simulink model "SWC_HALOUT_type"  (R2021b)
settings: Solver=FixedStepDiscrete  StartTime=0.0  StopTime=10.0  FixedStep=0.005  RelTol=1e-3
values from neighbouring files (symbols this model uses):
  DTC_10020B = Simulink.Parameter    [DTC_Constant_Definition.m]
  DTC_10020C = Simulink.Parameter    [DTC_Constant_Definition.m]
  DTC_10020D = Simulink.Parameter    [DTC_Constant_Definition.m]
  DTC_10020E = Simulink.Parameter    [DTC_Constant_Definition.m]
  DTC_100210 = Simulink.Parameter    [DTC_Constant_Definition.m]
  DTC_100211 = Simulink.Parameter    [DTC_Constant_Definition.m]
  DTC_100212 = Simulink.Parameter    [DTC_Constant_Definition.m]
  DTC_100213 = Simulink.Parameter    [DTC_Constant_Definition.m]
  DTC_100214 = Simulink.Parameter    [DTC_Constant_Definition.m]
  DTC_100215 = Simulink.Parameter    [DTC_Constant_Definition.m]
  DTC_100216 = Simulink.Parameter    [DTC_Constant_Definition.m]
  DTC_100217 = Simulink.Parameter    [DTC_Constant_Definition.m]
  DTC_100218 = Simulink.Parameter    [DTC_Constant_Definition.m]
  DTC_100219 = Simulink.Parameter    [DTC_Constant_Definition.m]
  DTC_10021A = Simulink.Parameter    [DTC_Constant_Definition.m]
  DTC_10021B = Simulink.Parameter    [DTC_Constant_Definition.m]
  DTC_10021C = Simulink.Parameter    [DTC_Constant_Definition.m]
  DTC_10021D = Simulink.Parameter    [DTC_Constant_Definition.m]
  DTC_10021E = Simulink.Parameter    [DTC_Constant_Definition.m]
  DTC_100220 = Simulink.Parameter    [DTC_Constant_Definition.m]
  DTC_100221 = Simulink.Parameter    [DTC_Constant_Definition.m]
  DTC_100223 = Simulink.Parameter    [DTC_Constant_Definition.m]
  DTC_100224 = Simulink.Parameter    [DTC_Constant_Definition.m]
  DTC_100225 = Simulink.Parameter    [DTC_Constant_Definition.m]
  DTC_100226 = Simulink.Parameter    [DTC_Constant_Definition.m]
  DTC_100227 = Simulink.Parameter    [DTC_Constant_Definition.m]
  DTC_100242 = Simulink.Parameter    [DTC_Constant_Definition.m]
  DTC_100243 = Simulink.Parameter    [DTC_Constant_Definition.m]
  DTC_100244 = Simulink.Parameter    [DTC_Constant_Definition.m]
  DTC_100247 = Simulink.Parameter    [DTC_Constant_Definition.m]
  DTC_100248 = Simulink.Parameter    [DTC_Constant_Definition.m]
  DTC_100249 = Simulink.Parameter    [DTC_Constant_Definition.m]
  DTC_100250 = Simulink.Parameter    [DTC_Constant_Definition.m]
  DTC_100251 = Simulink.Parameter    [DTC_Constant_Definition.m]
  DTC_100252 = Simulink.Parameter    [DTC_Constant_Definition.m]
  DTC_100A10 = Simulink.Parameter    [DTC_Constant_Definition.m]
  DTC_100A12 = Simulink.Parameter    [DTC_Constant_Definition.m]
  DTC_100A16 = Simulink.Parameter    [DTC_Constant_Definition.m]
  DTC_100A17 = Simulink.Parameter    [DTC_Constant_Definition.m]
  DTC_100A18 = Simulink.Parameter    [DTC_Constant_Definition.m]
  DTC_100A19 = Simulink.Parameter    [DTC_Constant_Definition.m]
  DTC_500B01 = Simulink.Parameter    [DTC_Constant_Definition.m]
  DTC_500B02 = Simulink.Parameter    [DTC_Constant_Definition.m]
  DTC_500B03 = Simulink.Parameter    [DTC_Constant_Definition.m]
  DTC_500B04 = Simulink.Parameter    [DTC_Constant_Definition.m]
  DTC_500B05 = Simulink.Parameter    [DTC_Constant_Definition.m]
  DTC_500B06 = Simulink.Parameter    [DTC_Constant_Definition.m]
  DTC_500B07 = Simulink.Parameter    [DTC_Constant_Definition.m]
  DTC_500B08 = Simulink.Parameter    [DTC_Constant_Definition.m]
  DTC_500B09 = Simulink.Parameter    [DTC_Constant_Definition.m]
  DTC_500B0A = Simulink.Parameter    [DTC_Constant_Definition.m]
  DTC_500B0B = Simulink.Parameter    [DTC_Constant_Definition.m]
  DTC_500B0C = Simulink.Parameter    [DTC_Constant_Definition.m]
  DTC_500B0D = Simulink.Parameter    [DTC_Constant_Definition.m]
  DTC_500B0E = Simulink.Parameter    [DTC_Constant_Definition.m]
  DTC_500B0F = Simulink.Parameter    [DTC_Constant_Definition.m]
  DTC_500B10 = Simulink.Parameter    [DTC_Constant_Definition.m]
  DTC_90021F = Simulink.Parameter    [DTC_Constant_Definition.m]
  DTC_90022F = Simulink.Parameter    [DTC_Constant_Definition.m]
  DTC_900253 = Simulink.Parameter    [DTC_Constant_Definition.m]
  DTC_900254 = Simulink.Parameter    [DTC_Constant_Definition.m]
  DTC_900301 = Simulink.Parameter    [DTC_Constant_Definition.m]
  DTC_900302 = Simulink.Parameter    [DTC_Constant_Definition.m]
  DTC_900303 = Simulink.Parameter    [DTC_Constant_Definition.m]
  DTC_900304 = Simulink.Parameter    [DTC_Constant_Definition.m]
  DTC_900305 = Simulink.Parameter    [DTC_Constant_Definition.m]
  DTC_900909 = Simulink.Parameter    [DTC_Constant_Definition.m]
  DTC_90090A = Simulink.Parameter    [DTC_Constant_Definition.m]
  DTC_90090B = Simulink.Parameter    [DTC_Constant_Definition.m]
  DTC_90090C = Simulink.Parameter    [DTC_Constant_Definition.m]
  DTC_90090D = Simulink.Parameter    [DTC_Constant_Definition.m]
  DTC_90090E = Simulink.Parameter    [DTC_Constant_Definition.m]
  DTC_90090F = Simulink.Parameter    [DTC_Constant_Definition.m]
  DTC_900910 = Simulink.Parameter    [DTC_Constant_Definition.m]
  DTC_900911 = Simulink.Parameter    [DTC_Constant_Definition.m]
  DTC_900912 = Simulink.Parameter    [DTC_Constant_Definition.m]
  DTC_900913 = Simulink.Parameter    [DTC_Constant_Definition.m]
  DTC_900914 = Simulink.Parameter    [DTC_Constant_Definition.m]
  DTC_C0288F = Simulink.Parameter    [DTC_Constant_Definition.m]
  DTC_C0378F = Simulink.Parameter    [DTC_Constant_Definition.m]
  DTC_C0468F = Simulink.Parameter    [DTC_Constant_Definition.m]
  DTC_C0558F = Simulink.Parameter    [DTC_Constant_Definition.m]
  DTC_C0648F = Simulink.Parameter    [DTC_Constant_Definition.m]
  DTC_C0808F = Simulink.Parameter    [DTC_Constant_Definition.m]
  DTC_D00201 = Simulink.Parameter    [DTC_Constant_Definition.m]
  DTC_D00202 = Simulink.Parameter    [DTC_Constant_Definition.m]
  DTC_D00203 = Simulink.Parameter    [DTC_Constant_Definition.m]
  DTC_D00204 = Simulink.Parameter    [DTC_Constant_Definition.m]
  DTC_D00205 = Simulink.Parameter    [DTC_Constant_Definition.m]
  DTC_D00206 = Simulink.Parameter    [DTC_Constant_Definition.m]
  DTC_D00207 = Simulink.Parameter    [DTC_Constant_Definition.m]
  DTC_D00208 = Simulink.Parameter    [DTC_Constant_Definition.m]
  DTC_D00209 = Simulink.Parameter    [DTC_Constant_Definition.m]
  DTC_D0020A = Simulink.Parameter    [DTC_Constant_Definition.m]
  DTC_D00228 = Simulink.Parameter    [DTC_Constant_Definition.m]
  DTC_D00229 = Simulink.Parameter    [DTC_Constant_Definition.m]
  DTC_D0022A = Simulink.Parameter    [DTC_Constant_Definition.m]
  DTC_D0022B = Simulink.Parameter    [DTC_Constant_Definition.m]
  DTC_D0022C = Simulink.Parameter    [DTC_Constant_Definition.m]
  DTC_D0022D = Simulink.Parameter    [DTC_Constant_Definition.m]
  DTC_D00230 = Simulink.Parameter    [DTC_Constant_Definition.m]
  DTC_D00231 = Simulink.Parameter    [DTC_Constant_Definition.m]
  DTC_D00232 = Simulink.Parameter    [DTC_Constant_Definition.m]
  DTC_D00234 = Simulink.Parameter    [DTC_Constant_Definition.m]
  DTC_D00235 = Simulink.Parameter    [DTC_Constant_Definition.m]
  DTC_D00236 = Simulink.Parameter    [DTC_Constant_Definition.m]
  DTC_D00237 = Simulink.Parameter    [DTC_Constant_Definition.m]
  DTC_D00238 = Simulink.Parameter    [DTC_Constant_Definition.m]
  DTC_D0023A = Simulink.Parameter    [DTC_Constant_Definition.m]
  DTC_D0023B = Simulink.Parameter    [DTC_Constant_Definition.m]
  DTC_D0023C = Simulink.Parameter    [DTC_Constant_Definition.m]
  DTC_D0023D = Simulink.Parameter    [DTC_Constant_Definition.m]
  DTC_D0023E = Simulink.Parameter    [DTC_Constant_Definition.m]
  DTC_D00240 = Simulink.Parameter    [DTC_Constant_Definition.m]
  DTC_D00241 = Simulink.Parameter    [DTC_Constant_Definition.m]
undefined symbols (not defined in the file or in its folder): DIDLen_APPD, DIDLen_APPE, DIDLen_APPPedalZP, DIDLen_APSFunConfig, DIDLen_AutoLock, DIDLen_AutoWipHSpdEN, DIDLen_CALID, DIDLen_CDEODT, DIDLen_CLRDIST, DIDLen_DKCBLESta, DIDLen_DKCKey, DIDLen_DKCSta, DIDLen_DoorNFCAnchorSta, DIDLen_DRLDis, DIDLen_DynoMode, DIDLen_ECUNAME, DIDLen_FDDKCCoordXY, DIDLen_FMHTimer, DIDLen_LFLowPresThre, DIDLen_LFSensorID, DIDLen_LIDAAnchorSta, DIDLen_LRLowPresThre, DIDLen_LRSensorID, DIDLen_MILDIST, DIDLen_NUMPSATRIPSFLTMEMCLR, DIDLen_NVMPedalZP, DIDLen_OBDReq, DIDLen_ODOMETER, DIDLen_PKE, DIDLen_ProtocolId, DIDLen_PSA, DIDLen_QTYPSATRIPS, DIDLen_RFLowPresThre, DIDLen_RFSensorID, DIDLen_RRLowPresThre, DIDLen_RRSensorID, DIDLen_RUNTM, DIDLen_SensorMode, DIDLen_TestGroup, DIDLen_TireSize, DIDLen_TPMSLearnSta, DIDLen_UIDSta, DIDLen_USSConfig, DIDLen_UWBAnchorSta, DIDLen_VIN, DIDLen_VSS, DIDLen_WhlPres, DIDLen_WhlSensorBattSta, DIDLen_WhlTmp, DIDLen_WipRLSCmdCutFilter, DIDLen_WipRLSCmdHoldFilter, DIDLen_XWDMode, DIDNum_APPD, DIDNum_APPE, DIDNum_APPPedalZP, DIDNum_APSFunConfig, DIDNum_AutoLock, DIDNum_AutoWipHSpdEN, DIDNum_CALID, DIDNum_CDEODT ... (+281)
libraries: simulink x213, FVT_lib x160, hdlsllib x6, hcu_lib x5, halout x1
(part 1 of 9)
settings Model: DataDictionary=APPTypes.sldd  Creator=FVT23010  LastModifiedBy=FVT23033
settings DataIOCC: SaveFormat=StructureWithTime
settings OptimizationCC: DefaultParameterBehavior=Inlined  EnhancedBackFolding=on  PassReuseOutputArgsAs=Individual arguments  ZeroExternalMemoryAtStartup=off  ZeroInternalMemoryAtStartup=off  OptimizeBlockOrder=speed  DifferentSizesBufferReuse=on  OptimizationCustomize=off  EfficientTunableParamExpr=on
settings DebuggingCC: ParameterTunabilityLossMsg=error
settings HardwareCC: ProdBitPerPointer=32  ProdBitPerSizeT=32  ProdBitPerPtrDiffT=32  ProdLargestAtomicInteger=Long  ProdLargestAtomicFloat=Double  ProdWordSize=32  ProdLongLongMode=on  ProdHWDeviceType=ARM Compatible->ARM Cortex-M
settings ModelReferenceCC: ModelReferenceNumInstancesAllowed=Single
settings SFSimCC: MATLABDynamicMemAlloc=off
settings RTWCC: Description=AUTOSAR  SystemTargetFile=autosar.tlc  GenCodeOnly=on  TemplateMakefile=ert_default_tmf  PortableWordSizes=on
settings CodeAppCC: ForceParamTrailComments=on  IgnoreCustomStorageClasses=off  OperatorAnnotations=on  SimulinkDataObjDesc=on  SFDataObjDesc=on  InsertBlockDesc=on
settings STFCustomTargetCC: TargetLangStandard=C99 (ISO)  UtilityFuncGeneration=Shared location  MultiwordLength=256  ParMdlRefBuildCompliant=on  CompOptLevelCompliant=on  IncludeMdlTerminateFcn=off  CombineOutputUpdateFcns=on  SuppressErrorStatus=on  ERTCustomFileBanners=on  SupportNonFinite=off  SupportComplex=off  SupportContinuousTime=off  SupportNonInlinedSFcns=off  RemoveResetFunc=on  MATLABClassNameForMDSCustomization=Simulink.SoftwareTarget.ERTCustomization  AutosarCompliant=on  GRTInterface=off  UseToolchainInfoCompliant=on  GenerateSharedConstants=off  LookupTableObjectStructAxisOrder=2,1,3,4,...  LUTObjectStructOrderEvenSpacing=Size,Table,Breakpoints  SystemTargetFile=autosar.tlc
settings ERTTargetCC: TargetLangStandard=C99 (ISO)  UtilityFuncGeneration=Shared location  ConcurrentExecutionCompliant=off  IncludeMdlTerminateFcn=off  SuppressErrorStatus=on  SupportNonFinite=off  SupportComplex=off  ModelStepFunctionPrototypeControlCompliant=off  CPPClassGenCompliant=off  AutosarCompliant=on  GenerateSharedConstants=off  LookupTableObjectStructAxisOrder=2,1,3,4,...  LUTObjectStructOrderEvenSpacing=Size,Table,Breakpoints  GenerateASAP2=on  InlinedParameterPlacement=NonHierarchical  ERTCustomFileTemplate=example_file_process.tlc  ConvertIfToSwitch=off  SuppressUnreachableDefaultCases=off  BooleanTrueId=true_MatlabRTW  BooleanFalseId=false_MatlabRTW

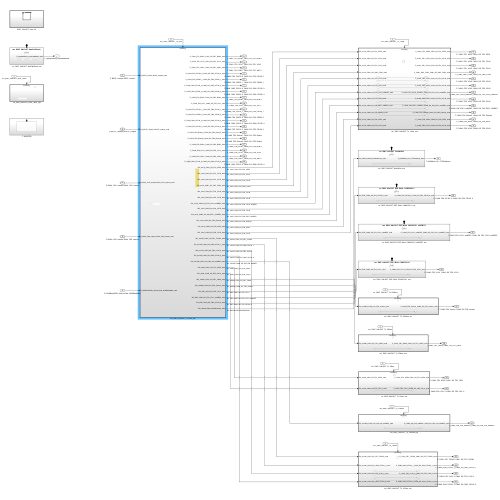
[thumbnail: Simulink's stored preview of the top-level diagram]
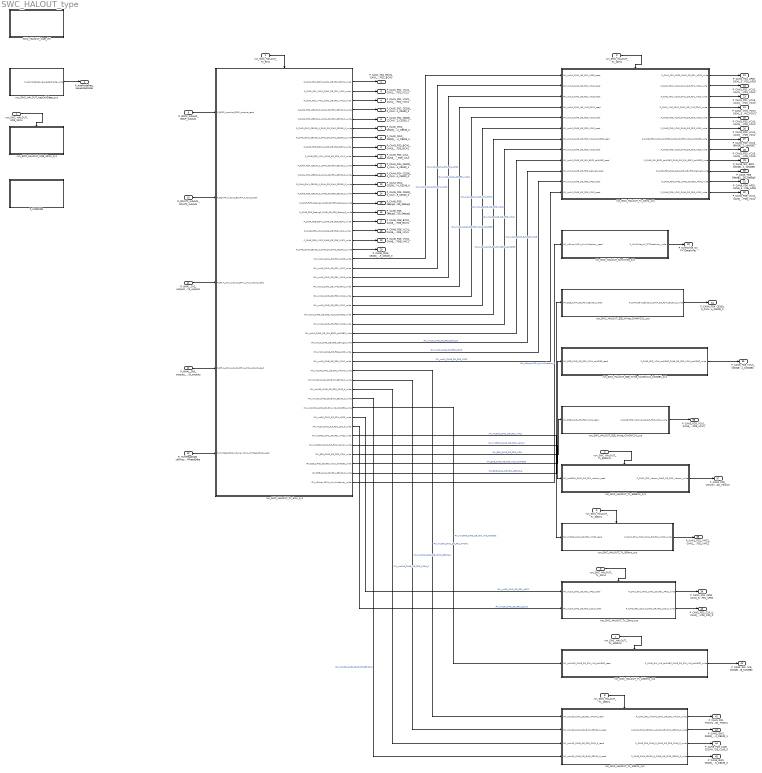
== system SWC_HALOUT_type ==
  run_SWC_HALOUT_UDS_10ms : Inport  SampleTime=0.01  OutputFunctionCall=on
  run_SWC_HALOUT_Tx_5ms : Inport  Port=2  SampleTime=0.005  OutputFunctionCall=on
  run_SWC_HALOUT_Tx_10ms : Inport  Port=3  SampleTime=0.01  OutputFunctionCall=on
  run_SWC_HALOUT_Tx_5000ms : Inport  Port=4  SampleTime=5  OutputFunctionCall=on
  run_SWC_HALOUT_Tx_500ms : Inport  Port=5  SampleTime=0.5  OutputFunctionCall=on
  run_SWC_HALOUT_Tx_20ms : Inport  Port=6  SampleTime=0.02  OutputFunctionCall=on
  run_SWC_HALOUT_Tx_1000ms : Inport  Port=7  SampleTime=1  OutputFunctionCall=on
  run_SWC_HALOUT_Tx_100ms : Inport  Port=8  SampleTime=0.1  OutputFunctionCall=on
  R_BSCP_outputs_BSCP_outputs : Inport  Port=9  OutDataTypeStr=Bus: BSCP_outputs  PortDimensions=1  BusOutputAsStruct=on
  R_BOUTP_outputs_BOUTP_outputs : Inport  Port=10  OutDataTypeStr=Bus: BOUTP_outputs  PortDimensions=1  BusOutputAsStruct=on
  R_BHAL_SYS_outputs_BHAL_SYS_outputs : Inport  Port=11  OutDataTypeStr=Bus: BHAL_SYS_outputs  PortDimensions=1  BusOutputAsStruct=on
  R_BHAL_DID_outputs_BHAL_DID_outputs : Inport  Port=12  OutDataTypeStr=Bus: BHAL_DID_outputs  PortDimensions=1  BusOutputAsStruct=on
  R_NVMReadCDD_u8Array1024_NVMReadData : Inport  Port=13  OutDataTypeStr=uint8  PortDimensions=1024
  P_WDGCDD : Subsystem
  SWC_HALOUT_type_Init : Subsystem
  run_SWC_HALOUT_AppCallSleep_sys : Subsystem
  run_SWC_HALOUT_E2E_Write_CAN3VCU1_sys : Subsystem
  run_SWC_HALOUT_E2E_Write_CAN3VCU1_toNIDEC_sys : Subsystem
  run_SWC_HALOUT_E2E_Write_CAN4VCU1_sys : Subsystem
  run_SWC_HALOUT_NvmWrite_sys : Subsystem
  run_SWC_HALOUT_Tx_1000ms_sys : Subsystem
  run_SWC_HALOUT_Tx_100ms_sys : Subsystem
  run_SWC_HALOUT_Tx_10ms_sys : Subsystem
  run_SWC_HALOUT_Tx_20ms_sys : Subsystem
  run_SWC_HALOUT_Tx_5000ms_sys : Subsystem
  run_SWC_HALOUT_Tx_500ms_sys : Subsystem
  run_SWC_HALOUT_Tx_5ms_sys : Subsystem
  run_SWC_HALOUT_UDS_10ms_sys : Subsystem
  P_AppModeReq_requestedMode : Outport  OutDataTypeStr=Enum: AppModeRequestType  PortDimensions=1
  P_CAN1_FD1_BCM1_CAN1_SG_FD1_BCM1 : Outport  Port=2  OutDataTypeStr=Bus: DT_CAN1_SG_FD1_BCM1  PortDimensions=1  BusOutputAsStruct=on
  P_CAN1_FD1_VCU1_CAN1_SG_FD1_VCU1 : Outport  Port=3  OutDataTypeStr=Bus: DT_CAN1_SG_FD1_VCU1  PortDimensions=1  BusOutputAsStruct=on
  P_CAN1_FD1_VMC1_CAN1_SG_FD1_VMC1 : Outport  Port=4  OutDataTypeStr=Bus: DT_CAN1_SG_FD1_VMC1  PortDimensions=1  BusOutputAsStruct=on
  P_CAN2_FD2_CE100_0_CAN2_SG_FD2_CE100_0 : Outport  Port=5  OutDataTypeStr=Bus: DT_CAN2_SG_FD2_CE100_0  PortDimensions=1  BusOutputAsStruct=on
  P_CAN2_FD2_CE200_1_CAN2_SG_FD2_CE200_1 : Outport  Port=6  OutDataTypeStr=Bus: DT_CAN2_SG_FD2_CE200_1  PortDimensions=1  BusOutputAsStruct=on
  P_CAN2_GW2_CE100_0_CAN2_SG_GW2_CE100_0 : Outport  Port=7  OutDataTypeStr=Bus: DT_CAN2_SG_GW2_CE100_0  PortDimensions=1  BusOutputAsStruct=on
  P_CAN2_GW2_CE200_0_CAN2_SG_GW2_CE200_0 : Outport  Port=8  OutDataTypeStr=Bus: DT_CAN2_SG_GW2_CE200_0  PortDimensions=1  BusOutputAsStruct=on
  P_CAN3_FD3_BCM1_CAN3_SG_FD3_BCM1 : Outport  Port=9  OutDataTypeStr=Bus: DT_CAN3_SG_FD3_BCM1  PortDimensions=1  BusOutputAsStruct=on
  P_CAN3_FD3_V2L1_CAN3_SG_FD3_V2L1 : Outport  Port=10  OutDataTypeStr=Bus: DT_CAN3_SG_FD3_V2L1  PortDimensions=1  BusOutputAsStruct=on
  P_CAN4_FD4_CE100_1_CAN4_SG_FD4_CE100_1 : Outport  Port=11  OutDataTypeStr=Bus: DT_CAN4_SG_FD4_CE100_1  PortDimensions=1  BusOutputAsStruct=on
  P_CAN4_FD4_CE200_0_CAN4_SG_FD4_CE200_0 : Outport  Port=12  OutDataTypeStr=Bus: DT_CAN4_SG_FD4_CE200_0  PortDimensions=1  BusOutputAsStruct=on
  P_CAN4_GW4_CE100_0_CAN4_SG_GW4_CE100_0 : Outport  Port=13  OutDataTypeStr=Bus: DT_CAN4_SG_GW4_CE100_0  PortDimensions=1  BusOutputAsStruct=on
  P_CAN5_FD5_CE100_0_CAN5_SG_FD5_CE100_0 : Outport  Port=14  OutDataTypeStr=Bus: DT_CAN5_SG_FD5_CE100_0  PortDimensions=1  BusOutputAsStruct=on
  P_CAN5_FD5_Debug1_CAN5_SG_FD5_Debug1 : Outport  Port=15  OutDataTypeStr=Bus: DT_CAN5_SG_FD5_Debug1  PortDimensions=1  BusOutputAsStruct=on
  P_CAN5_FD5_Debug2_CAN5_SG_FD5_Debug2 : Outport  Port=16  OutDataTypeStr=Bus: DT_CAN5_SG_FD5_Debug2  PortDimensions=1  BusOutputAsStruct=on
  P_CAN6_FD6_BCM1_CAN6_SG_FD6_BCM1 : Outport  Port=17  OutDataTypeStr=Bus: DT_CAN6_SG_FD6_BCM1  PortDimensions=1  BusOutputAsStruct=on
  P_CAN6_FD6_VCU1_CAN6_SG_FD6_VCU1 : Outport  Port=18  OutDataTypeStr=Bus: DT_CAN6_SG_FD6_VCU1  PortDimensions=1  BusOutputAsStruct=on
  P_CAN6_FD6_VMC1_CAN6_SG_FD6_VMC1 : Outport  Port=19  OutDataTypeStr=Bus: DT_CAN6_SG_FD6_VMC1  PortDimensions=1  BusOutputAsStruct=on
  P_CAN6_GW6_CE100_0_CAN6_SG_GW6_CE100_0 : Outport  Port=20  OutDataTypeStr=Bus: DT_CAN6_SG_GW6_CE100_0  PortDimensions=1  BusOutputAsStruct=on
  P_CAN1_FD1_APS3_CAN1_SG_FD1_APS3 : Outport  Port=21  OutDataTypeStr=Bus: DT_CAN1_SG_FD1_APS3  PortDimensions=1  BusOutputAsStruct=on
  P_CAN1_FD1_VCU2_CAN1_SG_FD1_VCU2 : Outport  Port=22  OutDataTypeStr=Bus: DT_CAN1_SG_FD1_VCU2  PortDimensions=1  BusOutputAsStruct=on
  P_CAN1_FD1_VCU3_CAN1_SG_FD1_VCU3 : Outport  Port=23  OutDataTypeStr=Bus: DT_CAN1_SG_FD1_VCU3  PortDimensions=1  BusOutputAsStruct=on
  P_CAN1_VMC_FCM1_CAN1_SG_VMC_FCM1 : Outport  Port=24  OutDataTypeStr=Bus: DT_CAN1_SG_VMC_FCM1  PortDimensions=1  BusOutputAsStruct=on
  P_CAN3_FD3_VCU0_CAN3_SG_FD3_VCU0 : Outport  Port=25  OutDataTypeStr=Bus: DT_CAN3_SG_FD3_VCU0  PortDimensions=1  BusOutputAsStruct=on
  P_CAN3_FD3_VCU2_CAN3_SG_FD3_VCU2 : Outport  Port=26  OutDataTypeStr=Bus: DT_CAN3_SG_FD3_VCU2  PortDimensions=1  BusOutputAsStruct=on
  P_CAN3_FD3_VCU2_toNIDEC_CAN3_SG_FD3_VCU2_toNIDEC : Outport  Port=27  OutDataTypeStr=Bus: DT_CAN3_SG_FD3_VCU2_toNIDEC  PortDimensions=1  BusOutputAsStruct=on
  P_CAN3_FD3_VCU5_CAN3_SG_FD3_VCU5 : Outport  Port=28  OutDataTypeStr=Bus: DT_CAN3_SG_FD3_VCU5  PortDimensions=1  BusOutputAsStruct=on
  P_CAN3_GW_ESC1_toNIDEC_CAN3_SG_GW_ESC1_toNIDEC : Outport  Port=29  OutDataTypeStr=Bus: DT_CAN3_SG_GW_ESC1_toNIDEC  PortDimensions=1  BusOutputAsStruct=on
  P_CAN5_FD5_Debug3_CAN5_SG_FD5_Debug3 : Outport  Port=30  OutDataTypeStr=Bus: DT_CAN5_SG_FD5_Debug3  PortDimensions=1  BusOutputAsStruct=on
  P_CAN6_FD6_APS3_CAN6_SG_FD6_APS3 : Outport  Port=31  OutDataTypeStr=Bus: DT_CAN6_SG_FD6_APS3  PortDimensions=1  BusOutputAsStruct=on
  P_CAN6_FD6_VCU2_CAN6_SG_FD6_VCU2 : Outport  Port=32  OutDataTypeStr=Bus: DT_CAN6_SG_FD6_VCU2  PortDimensions=1  BusOutputAsStruct=on
  P_NVMWrite_NV_FVTDataArray : Outport  Port=33  OutDataTypeStr=uint8  PortDimensions=1024
  P_CAN4_FD4_CE100_0_CAN4_SG_FD4_CE100_0 : Outport  Port=34  OutDataTypeStr=Bus: DT_CAN4_SG_FD4_CE100_0  PortDimensions=1  BusOutputAsStruct=on
  P_CAN3_FD3_VCU1_toNIDEC_CAN3_SG_FD3_VCU1_toNIDEC : Outport  Port=35  OutDataTypeStr=Bus: DT_CAN3_SG_FD3_VCU1_toNIDEC  PortDimensions=1  BusOutputAsStruct=on
  P_CAN3_FD3_VCU1_CAN3_SG_FD3_VCU1 : Outport  Port=36  OutDataTypeStr=Bus: DT_CAN3_SG_FD3_VCU1  PortDimensions=1  BusOutputAsStruct=on
  P_CAN2_FD2_Version_CAN2_SG_FD2_Version : Outport  Port=37  OutDataTypeStr=Bus: DT_CAN2_SG_FD2_Version  PortDimensions=1  BusOutputAsStruct=on
  P_CAN1_FD1_VMC2_CAN1_SG_FD1_VMC2 : Outport  Port=38  OutDataTypeStr=Bus: DT_CAN1_SG_FD1_VMC2  PortDimensions=1  BusOutputAsStruct=on
  P_CAN1_FD1_APS2_CAN1_SG_FD1_APS2 : Outport  Port=39  OutDataTypeStr=Bus: DT_CAN1_SG_FD1_APS2  PortDimensions=1  BusOutputAsStruct=on
  P_CAN2_FD2_C20_0_CAN2_SG_FD2_C20_0 : Outport  Port=40  OutDataTypeStr=Bus: DT_CAN2_SG_FD2_C20_0  PortDimensions=1  BusOutputAsStruct=on
  P_CAN3_GW_IVI6_toNIDEC_CAN3_SG_GW_IVI6_toNIDEC : Outport  Port=41  OutDataTypeStr=Bus: DT_CAN3_SG_GW_IVI6_toNIDEC  PortDimensions=1  BusOutputAsStruct=on
  P_CAN1_FD1_THCM1_CAN1_SG_FD1_THCM1 : Outport  Port=42  OutDataTypeStr=Bus: DT_CAN1_SG_FD1_THCM1  PortDimensions=1  BusOutputAsStruct=on
  P_CAN2_GW2_CE100_1_CAN2_SG_GW2_CE100_1 : Outport  Port=43  OutDataTypeStr=Bus: DT_CAN2_SG_GW2_CE100_1  PortDimensions=1  BusOutputAsStruct=on
  P_CAN3_FD3_C100_0_CAN3_SG_FD3_C100_0 : Outport  Port=44  OutDataTypeStr=Bus: DT_CAN3_SG_FD3_C100_0  PortDimensions=1  BusOutputAsStruct=on
  P_CAN5_GW5_CE100_0_CAN5_SG_GW5_CE100_0 : Outport  Port=45  OutDataTypeStr=Bus: DT_CAN5_SG_GW5_CE100_0  PortDimensions=1  BusOutputAsStruct=on
  wires:
  run_SWC_HALOUT_AppCallSleep_sys/1(P_AppModeReq_requestedMode_write) -> P_AppModeReq_requestedMode/1
  R_BSCP_outputs_BSCP_outputs/1 -> run_SWC_HALOUT_Tx_5ms_sys/1(R_BSCP_outputs_BSCP_outputs_read)
  R_BOUTP_outputs_BOUTP_outputs/1 -> run_SWC_HALOUT_Tx_5ms_sys/2(R_BOUTP_outputs_BOUTP_outputs_read)
  R_BHAL_SYS_outputs_BHAL_SYS_outputs/1 -> run_SWC_HALOUT_Tx_5ms_sys/3(R_BHAL_SYS_outputs_BHAL_SYS_outputs_read)
  R_BHAL_DID_outputs_BHAL_DID_outputs/1 -> run_SWC_HALOUT_Tx_5ms_sys/4(R_BHAL_DID_outputs_BHAL_DID_outputs_read)
  R_NVMReadCDD_u8Array1024_NVMReadData/1 -> run_SWC_HALOUT_Tx_5ms_sys/5(R_NVMReadCDD_u8Array1024_NVMReadData_read)
  run_SWC_HALOUT_Tx_5ms_sys/1(P_CAN1_FD1_BCM1_CAN1_SG_FD1_BCM1_write) -> P_CAN1_FD1_BCM1_CAN1_SG_FD1_BCM1/1
  run_SWC_HALOUT_Tx_5ms_sys/2(P_CAN1_FD1_VCU1_CAN1_SG_FD1_VCU1_write) -> P_CAN1_FD1_VCU1_CAN1_SG_FD1_VCU1/1
  run_SWC_HALOUT_Tx_5ms_sys/3(P_CAN1_FD1_VMC1_CAN1_SG_FD1_VMC1_write) -> P_CAN1_FD1_VMC1_CAN1_SG_FD1_VMC1/1
  run_SWC_HALOUT_Tx_5ms_sys/4(P_CAN2_FD2_CE100_0_CAN2_SG_FD2_CE100_0_write) -> P_CAN2_FD2_CE100_0_CAN2_SG_FD2_CE100_0/1
  run_SWC_HALOUT_Tx_5ms_sys/5(P_CAN2_FD2_CE200_1_CAN2_SG_FD2_CE200_1_write) -> P_CAN2_FD2_CE200_1_CAN2_SG_FD2_CE200_1/1
  run_SWC_HALOUT_Tx_5ms_sys/6(P_CAN2_GW2_CE100_0_CAN2_SG_GW2_CE100_0_write) -> P_CAN2_GW2_CE100_0_CAN2_SG_GW2_CE100_0/1
  run_SWC_HALOUT_Tx_5ms_sys/7(P_CAN2_GW2_CE200_0_CAN2_SG_GW2_CE200_0_write) -> P_CAN2_GW2_CE200_0_CAN2_SG_GW2_CE200_0/1
  run_SWC_HALOUT_Tx_5ms_sys/8(P_CAN3_FD3_BCM1_CAN3_SG_FD3_BCM1_write) -> P_CAN3_FD3_BCM1_CAN3_SG_FD3_BCM1/1
  run_SWC_HALOUT_Tx_5ms_sys/9(P_CAN3_FD3_V2L1_CAN3_SG_FD3_V2L1_write) -> P_CAN3_FD3_V2L1_CAN3_SG_FD3_V2L1/1
  run_SWC_HALOUT_Tx_5ms_sys/10(P_CAN4_FD4_CE100_1_CAN4_SG_FD4_CE100_1_write) -> P_CAN4_FD4_CE100_1_CAN4_SG_FD4_CE100_1/1
  run_SWC_HALOUT_Tx_5ms_sys/11(P_CAN4_FD4_CE200_0_CAN4_SG_FD4_CE200_0_write) -> P_CAN4_FD4_CE200_0_CAN4_SG_FD4_CE200_0/1
  run_SWC_HALOUT_Tx_5ms_sys/12(P_CAN4_GW4_CE100_0_CAN4_SG_GW4_CE100_0_write) -> P_CAN4_GW4_CE100_0_CAN4_SG_GW4_CE100_0/1
  run_SWC_HALOUT_Tx_5ms_sys/13(P_CAN5_FD5_CE100_0_CAN5_SG_FD5_CE100_0_write) -> P_CAN5_FD5_CE100_0_CAN5_SG_FD5_CE100_0/1
  run_SWC_HALOUT_Tx_5ms_sys/14(P_CAN5_FD5_Debug1_CAN5_SG_FD5_Debug1_write) -> P_CAN5_FD5_Debug1_CAN5_SG_FD5_Debug1/1
  run_SWC_HALOUT_Tx_5ms_sys/15(P_CAN5_FD5_Debug2_CAN5_SG_FD5_Debug2_write) -> P_CAN5_FD5_Debug2_CAN5_SG_FD5_Debug2/1
  run_SWC_HALOUT_Tx_5ms_sys/16(P_CAN6_FD6_BCM1_CAN6_SG_FD6_BCM1_write) -> P_CAN6_FD6_BCM1_CAN6_SG_FD6_BCM1/1
  run_SWC_HALOUT_Tx_5ms_sys/17(P_CAN6_FD6_VCU1_CAN6_SG_FD6_VCU1_write) -> P_CAN6_FD6_VCU1_CAN6_SG_FD6_VCU1/1
  run_SWC_HALOUT_Tx_5ms_sys/18(P_CAN6_FD6_VMC1_CAN6_SG_FD6_VMC1_write) -> P_CAN6_FD6_VMC1_CAN6_SG_FD6_VMC1/1
  run_SWC_HALOUT_Tx_5ms_sys/19(P_CAN6_GW6_CE100_0_CAN6_SG_GW6_CE100_0_write) -> P_CAN6_GW6_CE100_0_CAN6_SG_GW6_CE100_0/1
  run_SWC_HALOUT_Tx_10ms_sys/1(P_CAN1_FD1_APS3_CAN1_SG_FD1_APS3_write) -> P_CAN1_FD1_APS3_CAN1_SG_FD1_APS3/1
  run_SWC_HALOUT_Tx_10ms_sys/2(P_CAN1_FD1_VCU2_CAN1_SG_FD1_VCU2_write) -> P_CAN1_FD1_VCU2_CAN1_SG_FD1_VCU2/1
  run_SWC_HALOUT_Tx_10ms_sys/3(P_CAN1_FD1_VCU3_CAN1_SG_FD1_VCU3_write) -> P_CAN1_FD1_VCU3_CAN1_SG_FD1_VCU3/1
  run_SWC_HALOUT_Tx_10ms_sys/4(P_CAN1_VMC_FCM1_CAN1_SG_VMC_FCM1_write) -> P_CAN1_VMC_FCM1_CAN1_SG_VMC_FCM1/1
  run_SWC_HALOUT_Tx_10ms_sys/5(P_CAN3_FD3_VCU0_CAN3_SG_FD3_VCU0_write) -> P_CAN3_FD3_VCU0_CAN3_SG_FD3_VCU0/1
  run_SWC_HALOUT_Tx_10ms_sys/6(P_CAN3_FD3_VCU2_CAN3_SG_FD3_VCU2_write) -> P_CAN3_FD3_VCU2_CAN3_SG_FD3_VCU2/1
  run_SWC_HALOUT_Tx_10ms_sys/7(P_CAN3_FD3_VCU2_toNIDEC_CAN3_SG_FD3_VCU2_toNIDEC_write) -> P_CAN3_FD3_VCU2_toNIDEC_CAN3_SG_FD3_VCU2_toNIDEC/1
  run_SWC_HALOUT_Tx_10ms_sys/8(P_CAN3_FD3_VCU5_CAN3_SG_FD3_VCU5_write) -> P_CAN3_FD3_VCU5_CAN3_SG_FD3_VCU5/1
  run_SWC_HALOUT_Tx_10ms_sys/9(P_CAN3_GW_ESC1_toNIDEC_CAN3_SG_GW_ESC1_toNIDEC_write) -> P_CAN3_GW_ESC1_toNIDEC_CAN3_SG_GW_ESC1_toNIDEC/1
  run_SWC_HALOUT_Tx_10ms_sys/10(P_CAN5_FD5_Debug3_CAN5_SG_FD5_Debug3_write) -> P_CAN5_FD5_Debug3_CAN5_SG_FD5_Debug3/1
  run_SWC_HALOUT_Tx_10ms_sys/11(P_CAN6_FD6_APS3_CAN6_SG_FD6_APS3_write) -> P_CAN6_FD6_APS3_CAN6_SG_FD6_APS3/1
  run_SWC_HALOUT_Tx_10ms_sys/12(P_CAN6_FD6_VCU2_CAN6_SG_FD6_VCU2_write) -> P_CAN6_FD6_VCU2_CAN6_SG_FD6_VCU2/1
  run_SWC_HALOUT_NvmWrite_sys/1(P_NVMWrite_NV_FVTDataArray_write) -> P_NVMWrite_NV_FVTDataArray/1
  run_SWC_HALOUT_E2E_Write_CAN4VCU1_sys/1(P_CAN4_FD4_CE100_0_CAN4_SG_FD4_CE100_0_write) -> P_CAN4_FD4_CE100_0_CAN4_SG_FD4_CE100_0/1
  run_SWC_HALOUT_E2E_Write_CAN3VCU1_toNIDEC_sys/1(P_CAN3_FD3_VCU1_toNIDEC_CAN3_SG_FD3_VCU1_toNIDEC_write) -> P_CAN3_FD3_VCU1_toNIDEC_CAN3_SG_FD3_VCU1_toNIDEC/1
  run_SWC_HALOUT_E2E_Write_CAN3VCU1_sys/1(P_CAN3_FD3_VCU1_CAN3_SG_FD3_VCU1_write) -> P_CAN3_FD3_VCU1_CAN3_SG_FD3_VCU1/1
  run_SWC_HALOUT_Tx_5000ms_sys/1(P_CAN2_FD2_Version_CAN2_SG_FD2_Version_write) -> P_CAN2_FD2_Version_CAN2_SG_FD2_Version/1
  run_SWC_HALOUT_Tx_500ms_sys/1(P_CAN1_FD1_VMC2_CAN1_SG_FD1_VMC2_write) -> P_CAN1_FD1_VMC2_CAN1_SG_FD1_VMC2/1
  run_SWC_HALOUT_Tx_20ms_sys/1(P_CAN1_FD1_APS2_CAN1_SG_FD1_APS2_write) -> P_CAN1_FD1_APS2_CAN1_SG_FD1_APS2/1
  run_SWC_HALOUT_Tx_20ms_sys/2(P_CAN2_FD2_C20_0_CAN2_SG_FD2_C20_0_write) -> P_CAN2_FD2_C20_0_CAN2_SG_FD2_C20_0/1
  run_SWC_HALOUT_Tx_1000ms_sys/1(P_CAN3_GW_IVI6_toNIDEC_CAN3_SG_GW_IVI6_toNIDEC_write) -> P_CAN3_GW_IVI6_toNIDEC_CAN3_SG_GW_IVI6_toNIDEC/1
  run_SWC_HALOUT_Tx_100ms_sys/1(P_CAN1_FD1_THCM1_CAN1_SG_FD1_THCM1_write) -> P_CAN1_FD1_THCM1_CAN1_SG_FD1_THCM1/1
  run_SWC_HALOUT_Tx_100ms_sys/2(P_CAN2_GW2_CE100_1_CAN2_SG_GW2_CE100_1_write) -> P_CAN2_GW2_CE100_1_CAN2_SG_GW2_CE100_1/1
  run_SWC_HALOUT_Tx_100ms_sys/3(P_CAN3_FD3_C100_0_CAN3_SG_FD3_C100_0_write) -> P_CAN3_FD3_C100_0_CAN3_SG_FD3_C100_0/1
  run_SWC_HALOUT_Tx_100ms_sys/4(P_CAN5_GW5_CE100_0_CAN5_SG_GW5_CE100_0_write) -> P_CAN5_GW5_CE100_0_CAN5_SG_GW5_CE100_0/1
  run_SWC_HALOUT_Tx_5ms_sys/20(IRV_ms10_CAN1_SG_FD1_APS3_write) -> run_SWC_HALOUT_Tx_10ms_sys/1(IRV_ms10_CAN1_SG_FD1_APS3_read)  "IRV_ms10_CAN1_SG_FD1_APS3"
  run_SWC_HALOUT_Tx_5ms_sys/21(IRV_ms10_CAN1_SG_FD1_VCU2_write) -> run_SWC_HALOUT_Tx_10ms_sys/2(IRV_ms10_CAN1_SG_FD1_VCU2_read)  "IRV_ms10_CAN1_SG_FD1_VCU2"
  run_SWC_HALOUT_Tx_5ms_sys/22(IRV_ms10_CAN1_SG_FD1_VCU3_write) -> run_SWC_HALOUT_Tx_10ms_sys/3(IRV_ms10_CAN1_SG_FD1_VCU3_read)  "IRV_ms10_CAN1_SG_FD1_VCU3"
  run_SWC_HALOUT_Tx_5ms_sys/23(IRV_ms10_CAN1_SG_VMC_FCM1_write) -> run_SWC_HALOUT_Tx_10ms_sys/4(IRV_ms10_CAN1_SG_VMC_FCM1_read)  "IRV_ms10_CAN1_SG_VMC_FCM1"
  run_SWC_HALOUT_Tx_5ms_sys/24(IRV_ms10_CAN3_SG_FD3_VCU0_write) -> run_SWC_HALOUT_Tx_10ms_sys/5(IRV_ms10_CAN3_SG_FD3_VCU0_read)  "IRV_ms10_CAN3_SG_FD3_VCU0"
  run_SWC_HALOUT_Tx_5ms_sys/25(IRV_ms10_CAN3_SG_FD3_VCU2_write) -> run_SWC_HALOUT_Tx_10ms_sys/6(IRV_ms10_CAN3_SG_FD3_VCU2_read)  "IRV_ms10_CAN3_SG_FD3_VCU2"
  run_SWC_HALOUT_Tx_5ms_sys/26(IRV_ms10_CAN3_SG_FD3_VCU2_toNIDEC_write) -> run_SWC_HALOUT_Tx_10ms_sys/7(IRV_ms10_CAN3_SG_FD3_VCU2_toNIDEC_read)  "IRV_ms10_CAN3_SG_FD3_VCU2_toNIDEC"
  run_SWC_HALOUT_Tx_5ms_sys/27(IRV_ms10_CAN3_SG_FD3_VCU5_write) -> run_SWC_HALOUT_Tx_10ms_sys/8(IRV_ms10_CAN3_SG_FD3_VCU5_read)  "IRV_ms10_CAN3_SG_FD3_VCU5"
  run_SWC_HALOUT_Tx_5ms_sys/28(IRV_ms10_CAN3_SG_GW_ESC1_toNIDEC_write) -> run_SWC_HALOUT_Tx_10ms_sys/9(IRV_ms10_CAN3_SG_GW_ESC1_toNIDEC_read)  "IRV_ms10_CAN3_SG_GW_ESC1_toNIDEC"
  run_SWC_HALOUT_Tx_5ms_sys/29(IRV_ms10_CAN5_SG_FD5_Debug3_write) -> run_SWC_HALOUT_Tx_10ms_sys/10(IRV_ms10_CAN5_SG_FD5_Debug3_read)  "IRV_ms10_CAN5_SG_FD5_Debug3"
  run_SWC_HALOUT_Tx_5ms_sys/30(IRV_ms10_CAN6_SG_FD6_APS3_write) -> run_SWC_HALOUT_Tx_10ms_sys/11(IRV_ms10_CAN6_SG_FD6_APS3_read)  "IRV_ms10_CAN6_SG_FD6_APS3"
  run_SWC_HALOUT_Tx_5ms_sys/31(IRV_ms10_CAN6_SG_FD6_VCU2_write) -> run_SWC_HALOUT_Tx_10ms_sys/12(IRV_ms10_CAN6_SG_FD6_VCU2_read)  "IRV_ms10_CAN6_SG_FD6_VCU2"
  run_SWC_HALOUT_Tx_5ms_sys/32(IRV_ms100_CAN1_SG_FD1_THCM1_write) -> run_SWC_HALOUT_Tx_100ms_sys/1(IRV_ms100_CAN1_SG_FD1_THCM1_read)  "IRV_ms100_CAN1_SG_FD1_THCM1"
  run_SWC_HALOUT_Tx_5ms_sys/33(IRV_ms100_CAN2_SG_GW2_CE100_1_write) -> run_SWC_HALOUT_Tx_100ms_sys/2(IRV_ms100_CAN2_SG_GW2_CE100_1_read)  "IRV_ms100_CAN2_SG_GW2_CE100_1"
  run_SWC_HALOUT_Tx_5ms_sys/34(IRV_ms100_CAN3_SG_FD3_C100_0_write) -> run_SWC_HALOUT_Tx_100ms_sys/3(IRV_ms100_CAN3_SG_FD3_C100_0_read)  "IRV_ms100_CAN3_SG_FD3_C100_0"
  run_SWC_HALOUT_Tx_5ms_sys/35(IRV_ms100_CAN5_SG_GW5_CE100_0_write) -> run_SWC_HALOUT_Tx_100ms_sys/4(IRV_ms100_CAN5_SG_GW5_CE100_0_read)  "IRV_ms100_CAN5_SG_GW5_CE100_0"
  run_SWC_HALOUT_Tx_5ms_sys/36(IRV_ms1000_CAN3_SG_GW_IVI6_toNIDEC_write) -> run_SWC_HALOUT_Tx_1000ms_sys/1(IRV_ms1000_CAN3_SG_GW_IVI6_toNIDEC_read)  "IRV_ms1000_CAN3_SG_GW_IVI6_toNIDEC"
  run_SWC_HALOUT_Tx_5ms_sys/37(IRV_ms20_CAN1_SG_FD1_APS2_write) -> run_SWC_HALOUT_Tx_20ms_sys/1(IRV_ms20_CAN1_SG_FD1_APS2_read)  "IRV_ms20_CAN1_SG_FD1_APS2"
  run_SWC_HALOUT_Tx_5ms_sys/38(IRV_ms20_CAN2_SG_FD2_C20_0_write) -> run_SWC_HALOUT_Tx_20ms_sys/2(IRV_ms20_CAN2_SG_FD2_C20_0_read)  "IRV_ms20_CAN2_SG_FD2_C20_0"
  run_SWC_HALOUT_Tx_5ms_sys/39(IRV_ms500_CAN1_SG_FD1_VMC2_write) -> run_SWC_HALOUT_Tx_500ms_sys/1(IRV_ms500_CAN1_SG_FD1_VMC2_read)  "IRV_ms500_CAN1_SG_FD1_VMC2"
  run_SWC_HALOUT_Tx_5ms_sys/40(IRV_ms5000_CAN2_SG_FD2_Version_write) -> run_SWC_HALOUT_Tx_5000ms_sys/1(IRV_ms5000_CAN2_SG_FD2_Version_read)  "IRV_ms5000_CAN2_SG_FD2_Version"
  run_SWC_HALOUT_Tx_5ms_sys/41(IRV_E2E_CAN3_SG_FD3_VCU1_write) -> run_SWC_HALOUT_E2E_Write_CAN3VCU1_sys/1(IRV_E2E_CAN3_SG_FD3_VCU1_read)  "IRV_E2E_CAN3_SG_FD3_VCU1"
  run_SWC_HALOUT_Tx_5ms_sys/42(IRV_E2E_CAN3_SG_FD3_VCU1_toNIDEC_write) -> run_SWC_HALOUT_E2E_Write_CAN3VCU1_toNIDEC_sys/1(IRV_E2E_CAN3_SG_FD3_VCU1_toNIDEC_read)  "IRV_E2E_CAN3_SG_FD3_VCU1_toNIDEC"
  run_SWC_HALOUT_Tx_5ms_sys/43(IRV_E2E_CAN4_SG_FD4_CE100_0_write) -> run_SWC_HALOUT_E2E_Write_CAN4VCU1_sys/1(IRV_E2E_CAN4_SG_FD4_CE100_0_read)  "IRV_E2E_CAN4_SG_FD4_CE100_0"
  run_SWC_HALOUT_Tx_5ms_sys/44(IRV_u8Array1024_NvmWriteArray_write) -> run_SWC_HALOUT_NvmWrite_sys/1(IRV_u8Array1024_NvmWriteArray_read)  "IRV_u8Array1024_NvmWriteArray"
  run_SWC_HALOUT_UDS_10ms/1 -> run_SWC_HALOUT_UDS_10ms_sys/Trigger
  run_SWC_HALOUT_Tx_5ms/1 -> run_SWC_HALOUT_Tx_5ms_sys/Trigger
  run_SWC_HALOUT_Tx_10ms/1 -> run_SWC_HALOUT_Tx_10ms_sys/Trigger
  run_SWC_HALOUT_Tx_5000ms/1 -> run_SWC_HALOUT_Tx_5000ms_sys/Trigger
  run_SWC_HALOUT_Tx_500ms/1 -> run_SWC_HALOUT_Tx_500ms_sys/Trigger
  run_SWC_HALOUT_Tx_20ms/1 -> run_SWC_HALOUT_Tx_20ms_sys/Trigger
  run_SWC_HALOUT_Tx_1000ms/1 -> run_SWC_HALOUT_Tx_1000ms_sys/Trigger
  run_SWC_HALOUT_Tx_100ms/1 -> run_SWC_HALOUT_Tx_100ms_sys/Trigger

== system SWC_HALOUT_type/P_WDGCDD ==
  run_SWC_HALOUT_AppCallWDG_End_sys : Subsystem

== system SWC_HALOUT_type/SWC_HALOUT_type_Init ==
  Event Listener : EventListener  EventName=reset

== system SWC_HALOUT_type/run_SWC_HALOUT_AppCallSleep_sys ==
  function : TriggerPort  TriggerType=function-call  IsSimulinkFunction=on  FunctionName=run_SWC_HALOUT_AppCallSleep  VariantControl=(inherit)
  Constant : Constant  Value=TRUE
  Data Type Conversion : DataTypeConversion  OutDataTypeStr=Enum: AppModeRequestType
  Data Type Conversion1 : DataTypeConversion  OutDataTypeStr=uint8
  P_AppModeReq_requestedMode_write : Outport
  wires:
  Data Type Conversion/1 -> P_AppModeReq_requestedMode_write/1
  Data Type Conversion1/1 -> Data Type Conversion/1
  Constant/1 -> Data Type Conversion1/1

== system SWC_HALOUT_type/run_SWC_HALOUT_E2E_Write_CAN3VCU1_sys ==
  IRV_E2E_CAN3_SG_FD3_VCU1_read : Inport
  function : TriggerPort  TriggerType=function-call  IsSimulinkFunction=on  FunctionName=run_SWC_HALOUT_E2E_Write_CAN3VCU1  VariantControl=(inherit)
  P_CAN3_FD3_VCU1_CAN3_SG_FD3_VCU1_write : Outport
  wires:
  IRV_E2E_CAN3_SG_FD3_VCU1_read/1 -> P_CAN3_FD3_VCU1_CAN3_SG_FD3_VCU1_write/1

== system SWC_HALOUT_type/run_SWC_HALOUT_E2E_Write_CAN3VCU1_toNIDEC_sys ==
  IRV_E2E_CAN3_SG_FD3_VCU1_toNIDEC_read : Inport
  function : TriggerPort  TriggerType=function-call  IsSimulinkFunction=on  FunctionName=run_SWC_HALOUT_E2E_Write_CAN3VCU1_toNIDEC  VariantControl=(inherit)
  P_CAN3_FD3_VCU1_toNIDEC_CAN3_SG_FD3_VCU1_toNIDEC_write : Outport
  wires:
  IRV_E2E_CAN3_SG_FD3_VCU1_toNIDEC_read/1 -> P_CAN3_FD3_VCU1_toNIDEC_CAN3_SG_FD3_VCU1_toNIDEC_write/1

== system SWC_HALOUT_type/run_SWC_HALOUT_E2E_Write_CAN4VCU1_sys ==
  IRV_E2E_CAN4_SG_FD4_CE100_0_read : Inport
  function : TriggerPort  TriggerType=function-call  IsSimulinkFunction=on  FunctionName=run_SWC_HALOUT_E2E_Write_CAN4VCU1  VariantControl=(inherit)
  P_CAN4_FD4_CE100_0_CAN4_SG_FD4_CE100_0_write : Outport
  wires:
  IRV_E2E_CAN4_SG_FD4_CE100_0_read/1 -> P_CAN4_FD4_CE100_0_CAN4_SG_FD4_CE100_0_write/1

== system SWC_HALOUT_type/run_SWC_HALOUT_NvmWrite_sys ==
  IRV_u8Array1024_NvmWriteArray_read : Inport
  function : TriggerPort  TriggerType=function-call  IsSimulinkFunction=on  FunctionName=run_SWC_HALOUT_NvmWrite  VariantControl=(inherit)
  P_NVMWrite_NV_FVTDataArray_write : Outport
  wires:
  IRV_u8Array1024_NvmWriteArray_read/1 -> P_NVMWrite_NV_FVTDataArray_write/1

== system SWC_HALOUT_type/run_SWC_HALOUT_Tx_1000ms_sys ==
  IRV_ms1000_CAN3_SG_GW_IVI6_toNIDEC_read : Inport
  function : TriggerPort  TriggerType=function-call  VariantControl=(inherit)  SampleTimeType=periodic  SampleTime=-1
  P_CAN3_GW_IVI6_toNIDEC_CAN3_SG_GW_IVI6_toNIDEC_write : Outport
  wires:
  IRV_ms1000_CAN3_SG_GW_IVI6_toNIDEC_read/1 -> P_CAN3_GW_IVI6_toNIDEC_CAN3_SG_GW_IVI6_toNIDEC_write/1

== system SWC_HALOUT_type/run_SWC_HALOUT_Tx_100ms_sys ==
  IRV_ms100_CAN1_SG_FD1_THCM1_read : Inport
  IRV_ms100_CAN2_SG_GW2_CE100_1_read : Inport  Port=2
  IRV_ms100_CAN3_SG_FD3_C100_0_read : Inport  Port=3
  IRV_ms100_CAN5_SG_GW5_CE100_0_read : Inport  Port=4
  function : TriggerPort  TriggerType=function-call  VariantControl=(inherit)  SampleTimeType=periodic  SampleTime=-1
  P_CAN1_FD1_THCM1_CAN1_SG_FD1_THCM1_write : Outport
  P_CAN2_GW2_CE100_1_CAN2_SG_GW2_CE100_1_write : Outport  Port=2
  P_CAN3_FD3_C100_0_CAN3_SG_FD3_C100_0_write : Outport  Port=3
  P_CAN5_GW5_CE100_0_CAN5_SG_GW5_CE100_0_write : Outport  Port=4
  wires:
  IRV_ms100_CAN1_SG_FD1_THCM1_read/1 -> P_CAN1_FD1_THCM1_CAN1_SG_FD1_THCM1_write/1
  IRV_ms100_CAN2_SG_GW2_CE100_1_read/1 -> P_CAN2_GW2_CE100_1_CAN2_SG_GW2_CE100_1_write/1
  IRV_ms100_CAN3_SG_FD3_C100_0_read/1 -> P_CAN3_FD3_C100_0_CAN3_SG_FD3_C100_0_write/1
  IRV_ms100_CAN5_SG_GW5_CE100_0_read/1 -> P_CAN5_GW5_CE100_0_CAN5_SG_GW5_CE100_0_write/1

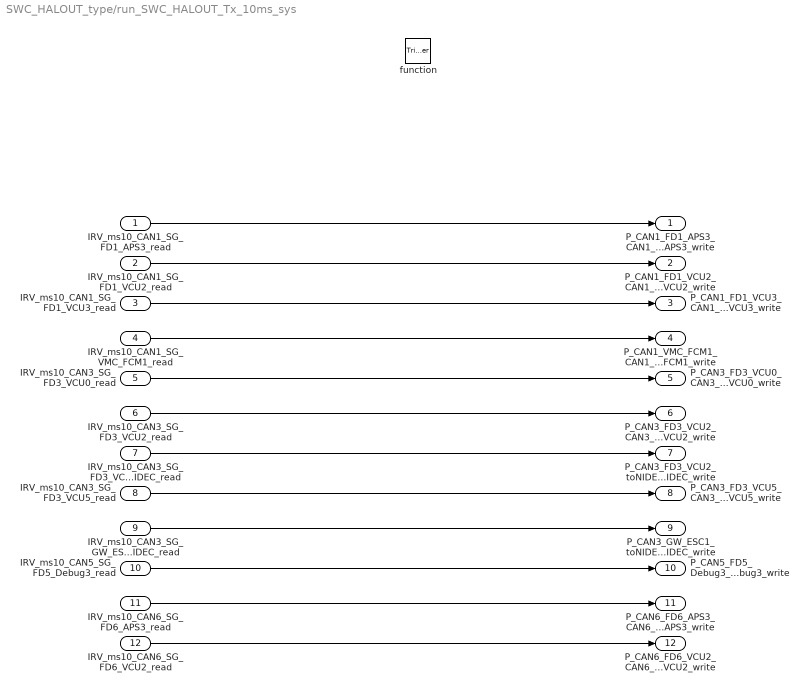
== system SWC_HALOUT_type/run_SWC_HALOUT_Tx_10ms_sys ==
  IRV_ms10_CAN1_SG_FD1_APS3_read : Inport
  IRV_ms10_CAN1_SG_FD1_VCU2_read : Inport  Port=2
  IRV_ms10_CAN1_SG_FD1_VCU3_read : Inport  Port=3
  IRV_ms10_CAN1_SG_VMC_FCM1_read : Inport  Port=4
  IRV_ms10_CAN3_SG_FD3_VCU0_read : Inport  Port=5
  IRV_ms10_CAN3_SG_FD3_VCU2_read : Inport  Port=6
  IRV_ms10_CAN3_SG_FD3_VCU2_toNIDEC_read : Inport  Port=7
  IRV_ms10_CAN3_SG_FD3_VCU5_read : Inport  Port=8
  IRV_ms10_CAN3_SG_GW_ESC1_toNIDEC_read : Inport  Port=9
  IRV_ms10_CAN5_SG_FD5_Debug3_read : Inport  Port=10
  IRV_ms10_CAN6_SG_FD6_APS3_read : Inport  Port=11
  IRV_ms10_CAN6_SG_FD6_VCU2_read : Inport  Port=12
  function : TriggerPort  TriggerType=function-call  VariantControl=(inherit)  SampleTimeType=periodic  SampleTime=-1
  P_CAN1_FD1_APS3_CAN1_SG_FD1_APS3_write : Outport
  P_CAN1_FD1_VCU2_CAN1_SG_FD1_VCU2_write : Outport  Port=2
  P_CAN1_FD1_VCU3_CAN1_SG_FD1_VCU3_write : Outport  Port=3
  P_CAN1_VMC_FCM1_CAN1_SG_VMC_FCM1_write : Outport  Port=4
  P_CAN3_FD3_VCU0_CAN3_SG_FD3_VCU0_write : Outport  Port=5
  P_CAN3_FD3_VCU2_CAN3_SG_FD3_VCU2_write : Outport  Port=6
  P_CAN3_FD3_VCU2_toNIDEC_CAN3_SG_FD3_VCU2_toNIDEC_write : Outport  Port=7
  P_CAN3_FD3_VCU5_CAN3_SG_FD3_VCU5_write : Outport  Port=8
  P_CAN3_GW_ESC1_toNIDEC_CAN3_SG_GW_ESC1_toNIDEC_write : Outport  Port=9
  P_CAN5_FD5_Debug3_CAN5_SG_FD5_Debug3_write : Outport  Port=10
  P_CAN6_FD6_APS3_CAN6_SG_FD6_APS3_write : Outport  Port=11
  P_CAN6_FD6_VCU2_CAN6_SG_FD6_VCU2_write : Outport  Port=12
  wires:
  IRV_ms10_CAN1_SG_FD1_APS3_read/1 -> P_CAN1_FD1_APS3_CAN1_SG_FD1_APS3_write/1
  IRV_ms10_CAN1_SG_FD1_VCU2_read/1 -> P_CAN1_FD1_VCU2_CAN1_SG_FD1_VCU2_write/1
  IRV_ms10_CAN1_SG_FD1_VCU3_read/1 -> P_CAN1_FD1_VCU3_CAN1_SG_FD1_VCU3_write/1
  IRV_ms10_CAN1_SG_VMC_FCM1_read/1 -> P_CAN1_VMC_FCM1_CAN1_SG_VMC_FCM1_write/1
  IRV_ms10_CAN3_SG_FD3_VCU0_read/1 -> P_CAN3_FD3_VCU0_CAN3_SG_FD3_VCU0_write/1
  IRV_ms10_CAN3_SG_FD3_VCU2_read/1 -> P_CAN3_FD3_VCU2_CAN3_SG_FD3_VCU2_write/1
  IRV_ms10_CAN3_SG_FD3_VCU2_toNIDEC_read/1 -> P_CAN3_FD3_VCU2_toNIDEC_CAN3_SG_FD3_VCU2_toNIDEC_write/1
  IRV_ms10_CAN3_SG_FD3_VCU5_read/1 -> P_CAN3_FD3_VCU5_CAN3_SG_FD3_VCU5_write/1
  IRV_ms10_CAN3_SG_GW_ESC1_toNIDEC_read/1 -> P_CAN3_GW_ESC1_toNIDEC_CAN3_SG_GW_ESC1_toNIDEC_write/1
  IRV_ms10_CAN5_SG_FD5_Debug3_read/1 -> P_CAN5_FD5_Debug3_CAN5_SG_FD5_Debug3_write/1
  IRV_ms10_CAN6_SG_FD6_APS3_read/1 -> P_CAN6_FD6_APS3_CAN6_SG_FD6_APS3_write/1
  IRV_ms10_CAN6_SG_FD6_VCU2_read/1 -> P_CAN6_FD6_VCU2_CAN6_SG_FD6_VCU2_write/1

== system SWC_HALOUT_type/run_SWC_HALOUT_Tx_20ms_sys ==
  IRV_ms20_CAN1_SG_FD1_APS2_read : Inport
  IRV_ms20_CAN2_SG_FD2_C20_0_read : Inport  Port=2
  function : TriggerPort  TriggerType=function-call  VariantControl=(inherit)  SampleTimeType=periodic  SampleTime=-1
  P_CAN1_FD1_APS2_CAN1_SG_FD1_APS2_write : Outport
  P_CAN2_FD2_C20_0_CAN2_SG_FD2_C20_0_write : Outport  Port=2
  wires:
  IRV_ms20_CAN1_SG_FD1_APS2_read/1 -> P_CAN1_FD1_APS2_CAN1_SG_FD1_APS2_write/1
  IRV_ms20_CAN2_SG_FD2_C20_0_read/1 -> P_CAN2_FD2_C20_0_CAN2_SG_FD2_C20_0_write/1

== system SWC_HALOUT_type/run_SWC_HALOUT_Tx_5000ms_sys ==
  IRV_ms5000_CAN2_SG_FD2_Version_read : Inport
  function : TriggerPort  TriggerType=function-call  VariantControl=(inherit)  SampleTimeType=periodic  SampleTime=-1
  P_CAN2_FD2_Version_CAN2_SG_FD2_Version_write : Outport
  wires:
  IRV_ms5000_CAN2_SG_FD2_Version_read/1 -> P_CAN2_FD2_Version_CAN2_SG_FD2_Version_write/1

== system SWC_HALOUT_type/run_SWC_HALOUT_Tx_500ms_sys ==
  IRV_ms500_CAN1_SG_FD1_VMC2_read : Inport
  function : TriggerPort  TriggerType=function-call  VariantControl=(inherit)  SampleTimeType=periodic  SampleTime=-1
  P_CAN1_FD1_VMC2_CAN1_SG_FD1_VMC2_write : Outport
  wires:
  IRV_ms500_CAN1_SG_FD1_VMC2_read/1 -> P_CAN1_FD1_VMC2_CAN1_SG_FD1_VMC2_write/1
